simulink model "ukl_reg_II"  (R2023a)
settings: Solver=VariableStepAuto  StartTime=0.0  StopTime=10.0  RelTol=1e-3
undefined symbols (not defined in the file): h, licz, mian3, ym
settings Model: Creator=jpawl  LastModifiedBy=jpawl

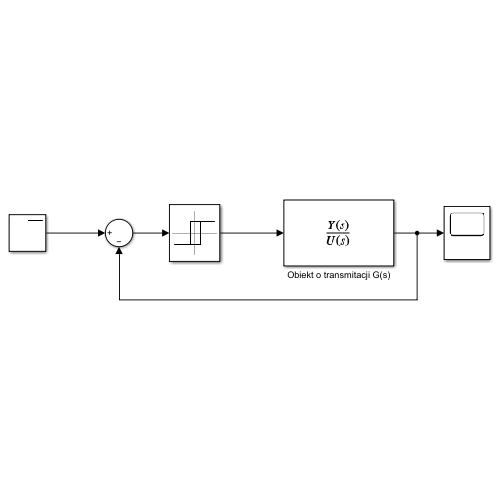
[thumbnail: Simulink's stored preview of the top-level diagram]
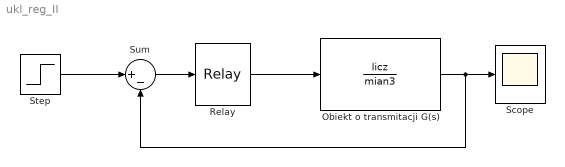
== system ukl_reg_II ==
  Obiekt o transmitacji G(s) : TransferFcn  Numerator=licz  Denominator=mian3
  Relay : Relay  OnSwitchValue=h  OffSwitchValue=-h  OnOutputValue=ym  OffOutputValue=-ym
  Scope : Scope
  Step : Step  SampleTime=0
  Sum : Sum  Inputs=|+-
  wires:
  Step/1 -> Sum/1
  Sum/1 -> Relay/1
  Relay/1 -> Obiekt o transmitacji G(s)/1
  Obiekt o transmitacji G(s)/1 -> Sum/2, Scope/1
